simulink model "exp2"  (R2023b)
settings: Solver=VariableStepAuto  StartTime=0.0  StopTime=10.0  RelTol=1e-3
libraries: commrandsrc3 x1

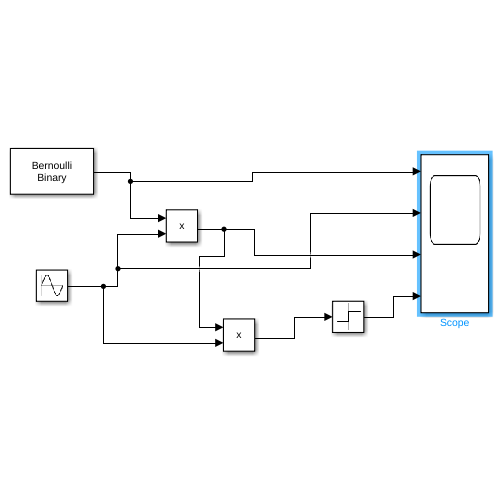
[thumbnail: Simulink's stored preview of the top-level diagram]
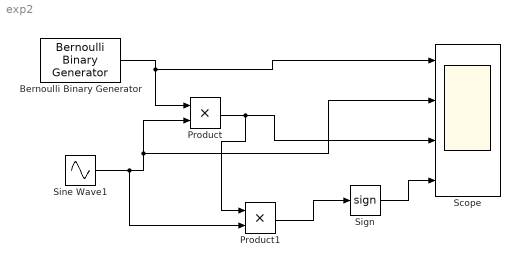
== system exp2 ==
  Bernoulli Binary Generator : commrandsrc3/Bernoulli Binary Generator  ProbabilityOfZero=0.5  SeedSource=Auto  Seed=0  SampleTime=1  SamplesPerFrame=1  OutputDataType=double  SimulateUsing=Interpreted execution
  Product : Product
  Product1 : Product
  Scope : Scope  NumInputPorts=4
  Sign : Signum
  Sine Wave1 : Sin  Frequency=2*pi*4  SampleTime=0
  wires:
  Bernoulli Binary Generator/1 -> Scope/1, Product/1
  Sine Wave1/1 -> Product1/2, Scope/2, Product/2
  Product/1 -> Product1/1, Scope/3
  Sign/1 -> Scope/4
  Product1/1 -> Sign/1
